simulink model "can_simple_block_bu11142"  (R2016b)
settings: Solver=FixedStepDiscrete  StartTime=0.0  StopTime=1000  FixedStep=0.2  RelTol=1e-3  EnableMultiTasking=on
undefined symbols (not defined in the file or in its folder): A, A10, A14, B, B11, B12, B13, B8, C, CS0, D, D11, D4, F3, F4, G3, G4, H3, H4, K17, K4, L3, N16, PA11, PA12, PD0, PE14, PE15, R10, R14, SCK, SIN, SOUT, T14
libraries: rappid_564xl_ec_toolbox x24
(part 2 of 2)

== stateflow chart can_simple_block_bu11142/Function-Call Subsystem/Data collection chart ==
  state Vol_C123
    en:
    CMD32[0] = 0x03;
    CMD32[1] = 0x70;
    CMD32[2] = 0x00;
    CMD32[3] = 0x04;
    STATE = 0;
    ex:
    Sig_Vol_C123;
  state GPIO45_Vref
    en:
    CMD32[0] = 0x04;
    CMD32[1] = 0x60;
    CMD32[2] = 0x00;
    CMD32[3] = 0x0E;
    STATE = 4;
    ex:
    Sig_GP45REF;
  state Vol_C456
    en:
    CMD32[0] = 0x03;
    CMD32[1] = 0x70;
    CMD32[2] = 0x00;
    CMD32[3] = 0x06;
    STATE = 1;
    ex:
    Sig_Vol_C456;
  state GPIO123
    en:
    CMD32[0] = 0x04;
    CMD32[1] = 0x60;
    CMD32[2] = 0x00;
    CMD32[3] = 0x0C;
    STATE = 3;
    ex:
    Sig_GP123;
  state Vol_C789
    en:
    CMD32[0] = 0x03;
    CMD32[1] = 0x70;
    CMD32[2] = 0x00;
    CMD32[3] = 0x08;
    STATE = 2;
    ex:
    Sig_Vol_C789;
  (default) -> Vol_C123 : {count =0;}
  GPIO45_Vref -> Vol_C123 : { count = count + 1;}
  GPIO123 -> GPIO45_Vref
  Vol_C123 -> Vol_C456
  Vol_C456 -> Vol_C789
  Vol_C789 -> GPIO123
  data: count output double [0..10000]; CMD32 output uint8 size=4; STATE output double
  events: Sig_Vol_C123 output FUNCTION_CALL_EVENT; Sig_GP123 output FUNCTION_CALL_EVENT; Sig_GP45REF output FUNCTION_CALL_EVENT; Sig_Vol_C456 output FUNCTION_CALL_EVENT; Sig_Vol_C789 output FUNCTION_CALL_EVENT

== matlab function can_simple_block_bu11142/Function-Call Subsystem/RawData to StoreData ==
  data: STATE input; SPIData input; PecChk input; CellV_1_104 data_store_memory; DataFault output
function DataFault   = fcn(STATE, SPIData, PecChk)

global CellV_1_104;
DataFault =  zeros(1,7);

switch STATE
  case 0 % VC123
    for i=1:7
      CellV_1_104(i*8-7) = uint16(SPIData(i*8-7))*256+uint16(SPIData(i*8-6));
      CellV_1_104(i*8-6) = uint16(SPIData(i*8-5))*256+uint16(SPIData(i*8-4));
      CellV_1_104(i*8-5) = uint16(SPIData(i*8-3))*256+uint16(SPIData(i*8-2));
      if (PecChk(i*2-1) == SPIData(i*8-1)) && (PecChk(i*2) == SPIData(i*8))
        DataFault(i) = 1;
      else
        DataFault(i) = 0;
      end
    end
  case 1 % VC456
    
  case 2 % VC78
    
  case 3 % GP123
    
  case 4 % GP45
    
  otherwise % ERROR
    
end








% CellV_1_104(1) = uint16(1);

% SPIDataStore = uint16(zeros(1,21));
% DataFault =  zeros(1,7);
% 
% for i=1:7
%   SPIDataStore(i*3-2) = SPIData(i*8-7)+SPIData(i*8-6)*256;
%   SPIDataStore(i*3-1) = SPIData(i*8-5)+SPIData(i*8-4)*256;
%   SPIDataStore(i*3   ) = SPIData(i*8-3)+SPIData(i*8-2)*256;
%   if (PecChk(i*2-1) == SPIData(i*8-1)) && (PecChk(i*2) == SPIData(i*8))
%     DataFault(i) = 1;
%   else
%     DataFault(i) = 0;
%   end
% end



% onemask8 = uint16(hex2dec('00FF'));
% onemask8_8sft = uint16(hex2dec('FF00'));
% onemask88 = uint8(hex2dec('FF'));
% onemask16 = uint16(hex2dec('FFFF'));
% 
% % data_test = zeros(1,2);
% remainder = uint16(16);
% 
% for i=1:len
%     ii = uint16(i);
% %     data_test(1,i) = data(ii);
% %     address = 2;
%     address = bitand( ...
%         bitxor( ...
%         uint8(bitsra(remainder,7)),data(ii) ), ...
%         onemask88);
%     remainder = bitxor(bitshift(remainder,8,'uint16'),pec15Table(address+1));
% end
% pec15 = uint16(bitand(bitshift(remainder,1,'uint16'),onemask16));
% pec0 = uint8(bitand(pec15,onemask8));
% pec1 = uint8(bitsra(bitand(pec15,onemask8_8sft),8));

== stateflow chart can_simple_block_bu11142/Function-Call Subsystem/Chart1 ==
  state A
    en: count = 0;
    du: count = count + 1;
  state A1
    en: count = 0;
  (default) -> A : {count =0;}
  A -> A1 : [count > count_in]{sig_trigger}
  A1 -> A
  data: count local double [0..10000]; count_in input
  events: sig_trigger output FUNCTION_CALL_EVENT

== matlab function can_simple_block_bu11142/Function-Call Subsystem/Subsystem/RawData to StoreData ==
  data: StrCell input; CellV_1_104 data_store_memory; VTDataCAN_8b output uint8
function VTDataCAN_8b = fcn(StrCell)

global CellV_1_104;
VTDataCAN_8b =  uint8(zeros(1,8));

      VTDataCAN_8b(1) =         CellV_1_104(StrCell*4-3)/256;
      VTDataCAN_8b(2) = mod(CellV_1_104(StrCell*4-3),256);
      VTDataCAN_8b(3) =         CellV_1_104(StrCell*4-2)/256;
      VTDataCAN_8b(4) = mod(CellV_1_104(StrCell*4-2),256);
      VTDataCAN_8b(5) =         CellV_1_104(StrCell*4-1)/256;
      VTDataCAN_8b(6) = mod(CellV_1_104(StrCell*4-1),256);
      VTDataCAN_8b(7) =         CellV_1_104(StrCell*4   )/256;
      VTDataCAN_8b(8) = mod(CellV_1_104(StrCell*4   ),256);

% VTDataCAN_8b(1) =         CellV_1_104(1)/256;
% VTDataCAN_8b(2) = mod(CellV_1_104(1),256);
% VTDataCAN_8b(3) =         CellV_1_104(2)/256;
% VTDataCAN_8b(4) = mod(CellV_1_104(2),256);
% VTDataCAN_8b(5) =         CellV_1_104(9)/256;
% VTDataCAN_8b(6) = mod(CellV_1_104(9),256);
% VTDataCAN_8b(7) =         CellV_1_104(10)/256;
% VTDataCAN_8b(8) = mod(CellV_1_104(10),256);

% VTDataCAN_8b(1) =         uint16(30000)/256;
% VTDataCAN_8b(2) = mod(uint16(30000),256);
% VTDataCAN_8b(3) =         uint16(35000)/256;
% VTDataCAN_8b(4) = mod(uint16(35000),256);
% VTDataCAN_8b(5) =         uint16(33000)/256;
% VTDataCAN_8b(6) = mod(uint16(33000),256);
% VTDataCAN_8b(7) =         uint16(20000)/256;
% VTDataCAN_8b(8) = mod(uint16(20000),256);


end








% CellV_1_104(1) = uint16(1);

% SPIDataStore = uint16(zeros(1,21));
% DataFault =  zeros(1,7);
%
% for i=1:7
%   SPIDataStore(i*3-2) = SPIData(i*8-7)+SPIData(i*8-6)*256;
%   SPIDataStore(i*3-1) = SPIData(i*8-5)+SPIData(i*8-4)*256;
%   SPIDataStore(i*3   ) = SPIData(i*8-3)+SPIData(i*8-2)*256;
%   if (PecChk(i*2-1) == SPIData(i*8-1)) && (PecChk(i*2) == SPIData(i*8))
%     DataFault(i) = 1;
%   else
%     DataFault(i) = 0;
%   end
% end



% onemask8 = uint16(hex2dec('00FF'));
% onemask8_8sft = uint16(hex2dec('FF00'));
% onemask88 = uint8(hex2dec('FF'));
% onemask16 = uint16(hex2dec('FFFF'));
%
% % data_test = zeros(1,2);
% remainder = uint16(16);
%
% for i=1:len
%     ii = uint16(i);
% %     data_test(1,i) = data(ii);
% %     address = 2;
%     address = bitand( ...
%         bitxor( ...
%         uint8(bitsra(remainder,7)),data(ii) ), ...
%         onemask88);
%     remainder = bitxor(bitshift(remainder,8,'uint16'),pec15Table(address+1));
% end
% pec15 = uint16(bitand(bitshift(remainder,1,'uint16'),onemask16));
% pec0 = uint8(bitand(pec15,onemask8));
% pec1 = uint8(bitsra(bitand(pec15,onemask8_8sft),8));

== stateflow chart can_simple_block_bu11142/Function-Call Subsystem/Subsystem/Chart1 ==
  state A
    en: count  = count + 1;
    du: count = count + 1;
  state A1
    en: count = 1;
  (default) -> A : {count =0;}
  A1 -> A
  A -> A1 : [count >= count_in]
  data: count_in input; count output double [0..10000]

== stateflow chart can_simple_block_bu11142/Function-Call Subsystem/Subsystem1/Chart1 ==
  state A
    en: count  = count + 1;
    du: count = count + 1;
  state A1
    en: count = 1;
  (default) -> A : {count =0;}
  A1 -> A
  A -> A1 : [count >= count_in]
  data: count_in input; count output double [0..10000]

== matlab function can_simple_block_bu11142/Function-Call Subsystem/Subsystem1/RawData to StoreData ==
  data: StrCell input; CellV_1_104 data_store_memory; VData_8 output uint8; TData output
function [VData_8,TData] = fcn(StrCell)

global CellV_1_104;
global CellGP_1_78;

VData_8 =  uint16(zeros(1,8));

VData_8(1) = CellV_1_104(StrCell*8-7);
VData_8(2) = CellV_1_104(StrCell*8-6);
VData_8(3) = CellV_1_104(StrCell*8-5);
VData_8(4) = CellV_1_104(StrCell*8-4);
VData_8(5) = CellV_1_104(StrCell*8-3);
VData_8(6) = CellV_1_104(StrCell*8-2);
VData_8(7) = CellV_1_104(StrCell*8-1);
VData_8(8) = CellV_1_104(StrCell*8   );
TData = 0.2*( CellGP_1_78(StrCell*5-4)+CellGP_1_78(StrCell*5-3) ...
  +CellGP_1_78(StrCell*5-2)+CellGP_1_78(StrCell*5-1)+CellGP_1_78(StrCell*5) );

% VTDataCAN_8b(1) =         CellV_1_104(1)/256;
% VTDataCAN_8b(2) = mod(CellV_1_104(1),256);
% VTDataCAN_8b(3) =         CellV_1_104(2)/256;
% VTDataCAN_8b(4) = mod(CellV_1_104(2),256);
% VTDataCAN_8b(5) =         CellV_1_104(9)/256;
% VTDataCAN_8b(6) = mod(CellV_1_104(9),256);
% VTDataCAN_8b(7) =         CellV_1_104(10)/256;
% VTDataCAN_8b(8) = mod(CellV_1_104(10),256);

% VTDataCAN_8b(1) =         uint16(30000)/256;
% VTDataCAN_8b(2) = mod(uint16(30000),256);
% VTDataCAN_8b(3) =         uint16(35000)/256;
% VTDataCAN_8b(4) = mod(uint16(35000),256);
% VTDataCAN_8b(5) =         uint16(33000)/256;
% VTDataCAN_8b(6) = mod(uint16(33000),256);
% VTDataCAN_8b(7) =         uint16(20000)/256;
% VTDataCAN_8b(8) = mod(uint16(20000),256);


end








% CellV_1_104(1) = uint16(1);

% SPIDataStore = uint16(zeros(1,21));
% DataFault =  zeros(1,7);
%
% for i=1:7
%   SPIDataStore(i*3-2) = SPIData(i*8-7)+SPIData(i*8-6)*256;
%   SPIDataStore(i*3-1) = SPIData(i*8-5)+SPIData(i*8-4)*256;
%   SPIDataStore(i*3   ) = SPIData(i*8-3)+SPIData(i*8-2)*256;
%   if (PecChk(i*2-1) == SPIData(i*8-1)) && (PecChk(i*2) == SPIData(i*8))
%     DataFault(i) = 1;
%   else
%     DataFault(i) = 0;
%   end
% end



% onemask8 = uint16(hex2dec('00FF'));
% onemask8_8sft = uint16(hex2dec('FF00'));
% onemask88 = uint8(hex2dec('FF'));
% onemask16 = uint16(hex2dec('FFFF'));
%
% % data_test = zeros(1,2);
% remainder = uint16(16);
%
% for i=1:len
%     ii = uint16(i);
% %     data_test(1,i) = data(ii);
% %     address = 2;
%     address = bitand( ...
%         bitxor( ...
%         uint8(bitsra(remainder,7)),data(ii) ), ...
%         onemask88);
%     remainder = bitxor(bitshift(remainder,8,'uint16'),pec15Table(address+1));
% end
% pec15 = uint16(bitand(bitshift(remainder,1,'uint16'),onemask16));
% pec0 = uint8(bitand(pec15,onemask8));
% pec1 = uint8(bitsra(bitand(pec15,onemask8_8sft),8));

== stateflow chart can_simple_block_bu11142/Function-Call Subsystem/Chart3 ==
  state InitDMA
    en: sig_DMAInit_trigger;
    du: count = count + 1;
  state DMA_Running
    en: count = 0;
  (default) -> InitDMA : {count =0;}
  InitDMA -> DMA_Running
  DMA_Running -> InitDMA : [DMA_RST == 1]
  data: count local double [0..10000]; count_in input; DMA_RST input
  events: sig_DMAInit_trigger output FUNCTION_CALL_EVENT

== stateflow chart can_simple_block_bu11142/Function-Call Subsystem/Chart4 ==
  state InitDMA
    en: sig_KFInit_trigger;
    du: count = count + 1;
  state DMA_Rest
    en: count = 0;
    du: count = count + 1;
  state DMA_Running
    en: count = 0;
  (default) -> InitDMA : {count =0;}
  InitDMA -> DMA_Rest
  DMA_Running -> InitDMA : [KF_RST == 1]
  DMA_Rest -> InitDMA [order 1] : [KF_RST == 1]
  DMA_Rest -> DMA_Running [order 2] : [count > count_in]{sig_KF_trigger}
  data: count local double [0..10000]; count_in input; KF_RST input
  events: sig_KFInit_trigger output FUNCTION_CALL_EVENT; sig_KF_trigger output FUNCTION_CALL_EVENT

== stateflow chart can_simple_block_bu11142/Function-Call Subsystem/SOCKF_Run/Chart1 ==
  state A
    en: count  = count + 1;
    du: count = count + 1;
  state A1
    en: count = 1;
  (default) -> A : {count =0;}
  A1 -> A
  A -> A1 : [count >= count_in]
  data: count_in input; count output double [0..10000]

== matlab function can_simple_block_bu11142/Function-Call Subsystem/SOCKF_Run/RawData to StoreData ==
  data: StrCell input; CellV_1_104 data_store_memory; VData_8 output uint16; TData output; CellGP_1_78 data_store_memory
function [VData_8,TData] = fcn(StrCell)

global CellV_1_104;
global CellGP_1_78;

VData_8 =  uint16(zeros(1,8));

VData_8(1) = CellV_1_104(StrCell*8-7);
VData_8(2) = CellV_1_104(StrCell*8-6);
VData_8(3) = CellV_1_104(StrCell*8-5);
VData_8(4) = CellV_1_104(StrCell*8-4);
VData_8(5) = CellV_1_104(StrCell*8-3);
VData_8(6) = CellV_1_104(StrCell*8-2);
VData_8(7) = CellV_1_104(StrCell*8-1);
VData_8(8) = CellV_1_104(StrCell*8   );
TData = 0.2*( CellGP_1_78(StrCell*5-4)+CellGP_1_78(StrCell*5-3) ...
  +CellGP_1_78(StrCell*5-2)+CellGP_1_78(StrCell*5-1)+CellGP_1_78(StrCell*5) );

% VTDataCAN_8b(1) =         CellV_1_104(1)/256;
% VTDataCAN_8b(2) = mod(CellV_1_104(1),256);
% VTDataCAN_8b(3) =         CellV_1_104(2)/256;
% VTDataCAN_8b(4) = mod(CellV_1_104(2),256);
% VTDataCAN_8b(5) =         CellV_1_104(9)/256;
% VTDataCAN_8b(6) = mod(CellV_1_104(9),256);
% VTDataCAN_8b(7) =         CellV_1_104(10)/256;
% VTDataCAN_8b(8) = mod(CellV_1_104(10),256);

% VTDataCAN_8b(1) =         uint16(30000)/256;
% VTDataCAN_8b(2) = mod(uint16(30000),256);
% VTDataCAN_8b(3) =         uint16(35000)/256;
% VTDataCAN_8b(4) = mod(uint16(35000),256);
% VTDataCAN_8b(5) =         uint16(33000)/256;
% VTDataCAN_8b(6) = mod(uint16(33000),256);
% VTDataCAN_8b(7) =         uint16(20000)/256;
% VTDataCAN_8b(8) = mod(uint16(20000),256);


end








% CellV_1_104(1) = uint16(1);

% SPIDataStore = uint16(zeros(1,21));
% DataFault =  zeros(1,7);
%
% for i=1:7
%   SPIDataStore(i*3-2) = SPIData(i*8-7)+SPIData(i*8-6)*256;
%   SPIDataStore(i*3-1) = SPIData(i*8-5)+SPIData(i*8-4)*256;
%   SPIDataStore(i*3   ) = SPIData(i*8-3)+SPIData(i*8-2)*256;
%   if (PecChk(i*2-1) == SPIData(i*8-1)) && (PecChk(i*2) == SPIData(i*8))
%     DataFault(i) = 1;
%   else
%     DataFault(i) = 0;
%   end
% end



% onemask8 = uint16(hex2dec('00FF'));
% onemask8_8sft = uint16(hex2dec('FF00'));
% onemask88 = uint8(hex2dec('FF'));
% onemask16 = uint16(hex2dec('FFFF'));
%
% % data_test = zeros(1,2);
% remainder = uint16(16);
%
% for i=1:len
%     ii = uint16(i);
% %     data_test(1,i) = data(ii);
% %     address = 2;
%     address = bitand( ...
%         bitxor( ...
%         uint8(bitsra(remainder,7)),data(ii) ), ...
%         onemask88);
%     remainder = bitxor(bitshift(remainder,8,'uint16'),pec15Table(address+1));
% end
% pec15 = uint16(bitand(bitshift(remainder,1,'uint16'),onemask16));
% pec0 = uint8(bitand(pec15,onemask8));
% pec1 = uint8(bitsra(bitand(pec15,onemask8_8sft),8));

== matlab function can_simple_block_bu11142/Function-Call Subsystem/SOCKF_Run/RawData to StoreData1 ==
  data: StrCell input; CellSOC_1_104 data_store_memory; SOCEsti input
function fcn(StrCell,SOCEsti)

global CellSOC_1_104;

      CellSOC_1_104(StrCell*8-7) = SOCEsti(1);
      CellSOC_1_104(StrCell*8-6) = SOCEsti(2);
      CellSOC_1_104(StrCell*8-5) = SOCEsti(3);
      CellSOC_1_104(StrCell*8-4) = SOCEsti(4);
      CellSOC_1_104(StrCell*8-3) = SOCEsti(5);
      CellSOC_1_104(StrCell*8-2) = SOCEsti(6);
      CellSOC_1_104(StrCell*8-1) = SOCEsti(7);
      CellSOC_1_104(StrCell*8-0) = SOCEsti(8);

end


% CellV_1_104(1) = uint16(1);

% SPIDataStore = uint16(zeros(1,21));
% DataFault =  zeros(1,7);
%
% for i=1:7
%   SPIDataStore(i*3-2) = SPIData(i*8-7)+SPIData(i*8-6)*256;
%   SPIDataStore(i*3-1) = SPIData(i*8-5)+SPIData(i*8-4)*256;
%   SPIDataStore(i*3   ) = SPIData(i*8-3)+SPIData(i*8-2)*256;
%   if (PecChk(i*2-1) == SPIData(i*8-1)) && (PecChk(i*2) == SPIData(i*8))
%     DataFault(i) = 1;
%   else
%     DataFault(i) = 0;
%   end
% end



% onemask8 = uint16(hex2dec('00FF'));
% onemask8_8sft = uint16(hex2dec('FF00'));
% onemask88 = uint8(hex2dec('FF'));
% onemask16 = uint16(hex2dec('FFFF'));
%
% % data_test = zeros(1,2);
% remainder = uint16(16);
%
% for i=1:len
%     ii = uint16(i);
% %     data_test(1,i) = data(ii);
% %     address = 2;
%     address = bitand( ...
%         bitxor( ...
%         uint8(bitsra(remainder,7)),data(ii) ), ...
%         onemask88);
%     remainder = bitxor(bitshift(remainder,8,'uint16'),pec15Table(address+1));
% end
% pec15 = uint16(bitand(bitshift(remainder,1,'uint16'),onemask16));
% pec0 = uint8(bitand(pec15,onemask8));
% pec1 = uint8(bitsra(bitand(pec15,onemask8_8sft),8));
